simulink model "snb_d"  (R2012b)
settings: Solver=FixedStepDiscrete  SolverMode=SingleTasking  StartTime=0.0  StopTime=10000  RelTol=1e-3
undefined symbols (not defined in the file): Down, pfb_coeff_gen_calc, Up, xlipgetpartsetting
libraries: xbsIndex_r4 x12106, casper_library_misc x14, casper_library_communications x8, casper_library_delays x1, xps_library x1
(part 20 of 79)

== system snb_d/ct/parity_check0 ==
  sync_in : Inport
  din : Inport  Port=2
  en : Inport  Port=3
  Delay : xbsIndex_r4/Delay  rst=off  infoeditControl=Selection of Reset will increase slice count due to use of real FFs and instead of SRLs  en=off  latency=1  dbl_ovrd=off  reg_retiming=on  block_type=delay
  Delay1 : xbsIndex_r4/Delay  rst=off  infoeditControl=Selection of Reset will increase slice count due to use of real FFs and instead of SRLs  en=off  latency=1  dbl_ovrd=off  reg_retiming=on  block_type=delay
  Delay2 : xbsIndex_r4/Delay  rst=off  infoeditControl=Selection of Reset will increase slice count due to use of real FFs and instead of SRLs  en=off  latency=1  dbl_ovrd=off  reg_retiming=on  block_type=delay
  Slice : xbsIndex_r4/Slice  nbits=64  boolean_output=off  mode=Lower Bit Location + Width  bit1=0  base1=MSB of Input  bit0=0  base0=LSB of Input  dbl_ovrd=off  block_type=slice
  Slice1 : xbsIndex_r4/Slice  nbits=1  boolean_output=off  mode=Upper Bit Location + Width  bit1=0  base1=MSB of Input  bit0=0  base0=LSB of Input  dbl_ovrd=off  block_type=slice
  bus_expand : Subsystem  AncestorBlock=casper_library_flow_control/bus_expand  mask(bus_expand){mode=divisions of equal size, outputNum=72, outputWidth=1, outputBinaryPt=0, outputArithmeticType=0, show_format=off, outputToWorkspace=off, variablePrefix=out, outputToModelAsWell=on}
      mask prompts: outputNum "Number of outputs:"; outputWidth "Output width:"; outputBinaryPt "Output binary point position:"; outputArithmeticType "Output arithmetic type (ufix=0, fix=1, bool=2):"; show_format "Print format string?"; outputToWorkspace "Output to workspace?"; variablePrefix "Variable name prefix:"; outputToModelAsWell "Output to model as well?"
      mask help:
      | Expands a 'bus' made using a bus_create or Xilinx
      | concat block.
      | The input will be divided into the specified number
      | of outputs with the specified arithmetic types.
      | Divisions are made from most significant bit.
      mask init: same as snb_d/bus_expand10
      settings: AttributesFormatString=72 outputs
      mask TypeOptions mode: divisions of equal size | divisions of arbitrary size
      mask Callback mode: bus_expand_callback();
      mask Callback outputWidth: bus_expand_callback();
      mask Callback outputToWorkspace: bus_expand_callback();
  parity : xbsIndex_r4/Logical  logical_function=XOR  inputs=72  en=off  latency=1  precision=Full  arith_type=Unsigned  n_bits=16  bin_pt=0  align_bp=on  dbl_ovrd=off  block_type=logical
  parity_error : xbsIndex_r4/Logical  logical_function=AND  inputs=2  en=off  latency=0  precision=Full  arith_type=Unsigned  n_bits=16  bin_pt=0  align_bp=on  dbl_ovrd=off  block_type=logical
  sync_out : Outport
  dout : Outport  Port=2
  dvalid : Outport  Port=3
  error : Outport  Port=4
  wires:
  Slice/1 -> dout/1
  parity_error/1 -> error/1
  parity/1 -> parity_error/1
  sync_in/1 -> Delay/1
  bus_expand/17(out56) -> parity/17
  bus_expand/9(out64) -> parity/9
  bus_expand/64(out9) -> parity/64
  bus_expand/25(out48) -> parity/25
  bus_expand/30(out43) -> parity/30
  bus_expand/39(out34) -> parity/39
  bus_expand/15(out58) -> parity/15
  bus_expand/23(out50) -> parity/23
  bus_expand/16(out57) -> parity/16
  bus_expand/56(out17) -> parity/56
  bus_expand/43(out30) -> parity/43
  bus_expand/34(out39) -> parity/34
  bus_expand/33(out40) -> parity/33
  bus_expand/55(out18) -> parity/55
  bus_expand/29(out44) -> parity/29
  bus_expand/42(out31) -> parity/42
  bus_expand/65(out8) -> parity/65
  bus_expand/10(out63) -> parity/10
  bus_expand/31(out42) -> parity/31
  bus_expand/6(out67) -> parity/6
  bus_expand/1(msb_out72) -> parity/1
  bus_expand/24(out49) -> parity/24
  bus_expand/28(out45) -> parity/28
  bus_expand/47(out26) -> parity/47
  bus_expand/63(out10) -> parity/63
  bus_expand/40(out33) -> parity/40
  bus_expand/20(out53) -> parity/20
  bus_expand/67(out6) -> parity/67
  bus_expand/72(lsb_out1) -> parity/72
  bus_expand/35(out38) -> parity/35
  bus_expand/45(out28) -> parity/45
  bus_expand/32(out41) -> parity/32
  bus_expand/57(out16) -> parity/57
  bus_expand/46(out27) -> parity/46
  bus_expand/38(out35) -> parity/38
  bus_expand/48(out25) -> parity/48
  bus_expand/68(out5) -> parity/68
  bus_expand/7(out66) -> parity/7
  bus_expand/27(out46) -> parity/27
  bus_expand/41(out32) -> parity/41
  bus_expand/62(out11) -> parity/62
  bus_expand/3(out70) -> parity/3
  bus_expand/70(out3) -> parity/70
  bus_expand/4(out69) -> parity/4
  bus_expand/37(out36) -> parity/37
  bus_expand/71(out2) -> parity/71
  bus_expand/19(out54) -> parity/19
  bus_expand/66(out7) -> parity/66
  bus_expand/8(out65) -> parity/8
  bus_expand/49(out24) -> parity/49
  bus_expand/50(out23) -> parity/50
  bus_expand/21(out52) -> parity/21
  bus_expand/60(out13) -> parity/60
  bus_expand/59(out14) -> parity/59
  bus_expand/12(out61) -> parity/12
  bus_expand/53(out20) -> parity/53
  bus_expand/69(out4) -> parity/69
  bus_expand/36(out37) -> parity/36
  bus_expand/13(out60) -> parity/13
  bus_expand/26(out47) -> parity/26
  bus_expand/51(out22) -> parity/51
  bus_expand/58(out15) -> parity/58
  bus_expand/61(out12) -> parity/61
  bus_expand/5(out68) -> parity/5
  bus_expand/44(out29) -> parity/44
  bus_expand/54(out19) -> parity/54
  bus_expand/18(out55) -> parity/18
  bus_expand/2(out71) -> parity/2
  bus_expand/22(out51) -> parity/22
  bus_expand/52(out21) -> parity/52
  bus_expand/14(out59) -> parity/14
  bus_expand/11(out62) -> parity/11
  Delay1/1 -> Slice/1
  en/1 -> Delay2/1
  Delay/1 -> sync_out/1
  din/1 -> bus_expand/1(bus_in), Delay1/1
  Delay2/1 -> dvalid/1, Slice1/1
  Slice1/1 -> parity_error/2

== system snb_d/ct/parity_check1 ==
  sync_in : Inport
  din : Inport  Port=2
  en : Inport  Port=3
  Delay : xbsIndex_r4/Delay  rst=off  infoeditControl=Selection of Reset will increase slice count due to use of real FFs and instead of SRLs  en=off  latency=1  dbl_ovrd=off  reg_retiming=on  block_type=delay
  Delay1 : xbsIndex_r4/Delay  rst=off  infoeditControl=Selection of Reset will increase slice count due to use of real FFs and instead of SRLs  en=off  latency=1  dbl_ovrd=off  reg_retiming=on  block_type=delay
  Delay2 : xbsIndex_r4/Delay  rst=off  infoeditControl=Selection of Reset will increase slice count due to use of real FFs and instead of SRLs  en=off  latency=1  dbl_ovrd=off  reg_retiming=on  block_type=delay
  Slice : xbsIndex_r4/Slice  nbits=64  boolean_output=off  mode=Lower Bit Location + Width  bit1=0  base1=MSB of Input  bit0=0  base0=LSB of Input  dbl_ovrd=off  block_type=slice
  Slice1 : xbsIndex_r4/Slice  nbits=1  boolean_output=off  mode=Upper Bit Location + Width  bit1=0  base1=MSB of Input  bit0=0  base0=LSB of Input  dbl_ovrd=off  block_type=slice
  bus_expand : Subsystem  AncestorBlock=casper_library_flow_control/bus_expand  mask(bus_expand){mode=divisions of equal size, outputNum=72, outputWidth=1, outputBinaryPt=0, outputArithmeticType=0, show_format=off, outputToWorkspace=off, variablePrefix=out, outputToModelAsWell=on}
      mask prompts: outputNum "Number of outputs:"; outputWidth "Output width:"; outputBinaryPt "Output binary point position:"; outputArithmeticType "Output arithmetic type (ufix=0, fix=1, bool=2):"; show_format "Print format string?"; outputToWorkspace "Output to workspace?"; variablePrefix "Variable name prefix:"; outputToModelAsWell "Output to model as well?"
      mask help:
      | Expands a 'bus' made using a bus_create or Xilinx
      | concat block.
      | The input will be divided into the specified number
      | of outputs with the specified arithmetic types.
      | Divisions are made from most significant bit.
      mask init: same as snb_d/bus_expand10
      settings: AttributesFormatString=72 outputs
      mask TypeOptions mode: divisions of equal size | divisions of arbitrary size
      mask Callback mode: bus_expand_callback();
      mask Callback outputWidth: bus_expand_callback();
      mask Callback outputToWorkspace: bus_expand_callback();
  parity : xbsIndex_r4/Logical  logical_function=XOR  inputs=72  en=off  latency=1  precision=Full  arith_type=Unsigned  n_bits=16  bin_pt=0  align_bp=on  dbl_ovrd=off  block_type=logical
  parity_error : xbsIndex_r4/Logical  logical_function=AND  inputs=2  en=off  latency=0  precision=Full  arith_type=Unsigned  n_bits=16  bin_pt=0  align_bp=on  dbl_ovrd=off  block_type=logical
  sync_out : Outport
  dout : Outport  Port=2
  dvalid : Outport  Port=3
  error : Outport  Port=4
  wires:
  Slice1/1 -> parity_error/2
  Delay2/1 -> Slice1/1, dvalid/1
  din/1 -> Delay1/1, bus_expand/1(bus_in)
  Delay/1 -> sync_out/1
  en/1 -> Delay2/1
  Delay1/1 -> Slice/1
  bus_expand/11(out62) -> parity/11
  bus_expand/14(out59) -> parity/14
  bus_expand/52(out21) -> parity/52
  bus_expand/22(out51) -> parity/22
  bus_expand/2(out71) -> parity/2
  bus_expand/18(out55) -> parity/18
  bus_expand/54(out19) -> parity/54
  bus_expand/44(out29) -> parity/44
  bus_expand/5(out68) -> parity/5
  bus_expand/61(out12) -> parity/61
  bus_expand/58(out15) -> parity/58
  bus_expand/51(out22) -> parity/51
  bus_expand/26(out47) -> parity/26
  bus_expand/13(out60) -> parity/13
  bus_expand/36(out37) -> parity/36
  bus_expand/69(out4) -> parity/69
  bus_expand/53(out20) -> parity/53
  bus_expand/12(out61) -> parity/12
  bus_expand/59(out14) -> parity/59
  bus_expand/60(out13) -> parity/60
  bus_expand/21(out52) -> parity/21
  bus_expand/50(out23) -> parity/50
  bus_expand/49(out24) -> parity/49
  bus_expand/8(out65) -> parity/8
  bus_expand/66(out7) -> parity/66
  bus_expand/19(out54) -> parity/19
  bus_expand/71(out2) -> parity/71
  bus_expand/37(out36) -> parity/37
  bus_expand/4(out69) -> parity/4
  bus_expand/70(out3) -> parity/70
  bus_expand/3(out70) -> parity/3
  bus_expand/62(out11) -> parity/62
  bus_expand/41(out32) -> parity/41
  bus_expand/27(out46) -> parity/27
  bus_expand/7(out66) -> parity/7
  bus_expand/68(out5) -> parity/68
  bus_expand/48(out25) -> parity/48
  bus_expand/38(out35) -> parity/38
  bus_expand/46(out27) -> parity/46
  bus_expand/57(out16) -> parity/57
  bus_expand/32(out41) -> parity/32
  bus_expand/45(out28) -> parity/45
  bus_expand/35(out38) -> parity/35
  bus_expand/72(lsb_out1) -> parity/72
  bus_expand/67(out6) -> parity/67
  bus_expand/20(out53) -> parity/20
  bus_expand/40(out33) -> parity/40
  bus_expand/63(out10) -> parity/63
  bus_expand/47(out26) -> parity/47
  bus_expand/28(out45) -> parity/28
  bus_expand/24(out49) -> parity/24
  bus_expand/1(msb_out72) -> parity/1
  bus_expand/6(out67) -> parity/6
  bus_expand/31(out42) -> parity/31
  bus_expand/10(out63) -> parity/10
  bus_expand/65(out8) -> parity/65
  bus_expand/42(out31) -> parity/42
  bus_expand/29(out44) -> parity/29
  bus_expand/55(out18) -> parity/55
  bus_expand/33(out40) -> parity/33
  bus_expand/34(out39) -> parity/34
  bus_expand/43(out30) -> parity/43
  bus_expand/56(out17) -> parity/56
  bus_expand/16(out57) -> parity/16
  bus_expand/23(out50) -> parity/23
  bus_expand/15(out58) -> parity/15
  bus_expand/39(out34) -> parity/39
  bus_expand/30(out43) -> parity/30
  bus_expand/25(out48) -> parity/25
  bus_expand/64(out9) -> parity/64
  bus_expand/9(out64) -> parity/9
  bus_expand/17(out56) -> parity/17
  sync_in/1 -> Delay/1
  parity/1 -> parity_error/1
  parity_error/1 -> error/1
  Slice/1 -> dout/1

== system snb_d/ct/parity_generation0 ==
  sync_in : Inport
  din : Inport  Port=2
  en : Inport  Port=3
  Concat : xbsIndex_r4/Concat  num_inputs=3  dbl_ovrd=off  block_type=concat
  Delay : xbsIndex_r4/Delay  rst=off  infoeditControl=Selection of Reset will increase slice count due to use of real FFs and instead of SRLs  en=off  latency=1  dbl_ovrd=off  reg_retiming=on  block_type=delay
  Delay1 : xbsIndex_r4/Delay  rst=off  infoeditControl=Selection of Reset will increase slice count due to use of real FFs and instead of SRLs  en=off  latency=1  dbl_ovrd=off  reg_retiming=on  block_type=delay
  Delay2 : xbsIndex_r4/Delay  rst=off  infoeditControl=Selection of Reset will increase slice count due to use of real FFs and instead of SRLs  en=off  latency=1  dbl_ovrd=off  reg_retiming=on  block_type=delay
  bus_expand : Subsystem  AncestorBlock=casper_library_flow_control/bus_expand  mask(bus_expand){mode=divisions of equal size, outputNum=64, outputWidth=1, outputBinaryPt=0, outputArithmeticType=0, show_format=off, outputToWorkspace=off, variablePrefix=out, outputToModelAsWell=on}
      mask prompts: outputNum "Number of outputs:"; outputWidth "Output width:"; outputBinaryPt "Output binary point position:"; outputArithmeticType "Output arithmetic type (ufix=0, fix=1, bool=2):"; show_format "Print format string?"; outputToWorkspace "Output to workspace?"; variablePrefix "Variable name prefix:"; outputToModelAsWell "Output to model as well?"
      mask help:
      | Expands a 'bus' made using a bus_create or Xilinx
      | concat block.
      | The input will be divided into the specified number
      | of outputs with the specified arithmetic types.
      | Divisions are made from most significant bit.
      mask init: same as snb_d/bus_expand10
      settings: AttributesFormatString=64 outputs
      mask TypeOptions mode: divisions of equal size | divisions of arbitrary size
      mask Callback mode: bus_expand_callback();
      mask Callback outputWidth: bus_expand_callback();
      mask Callback outputToWorkspace: bus_expand_callback();
  padding : xbsIndex_r4/Constant  const=0  gui_display_data_type=Fixed-point  arith_type=Unsigned  n_bits=72-64-1  bin_pt=0  preci_type=Single  exp_width=8  frac_width=24  explicit_period=on  period=1  equ=P=C  opselect=C  inp2=PCIN>>17  opr=+  inp1=P  carry=CIN  dbl_ovrd=off  block_type=constant
  parity : xbsIndex_r4/Logical  logical_function=XOR  inputs=64  en=off  latency=1  precision=Full  arith_type=Unsigned  n_bits=16  bin_pt=0  align_bp=on  dbl_ovrd=off  block_type=logical
  sync_out : Outport
  dout : Outport  Port=2
  dvalid : Outport  Port=3
  wires:
  padding/1 -> Concat/2
  Delay2/1 -> dvalid/1
  Concat/1 -> dout/1
  parity/1 -> Concat/1
  Delay1/1 -> Concat/3
  en/1 -> Delay2/1
  din/1 -> Delay1/1, bus_expand/1(bus_in)
  Delay/1 -> sync_out/1
  sync_in/1 -> Delay/1
  bus_expand/33(out32) -> parity/33
  bus_expand/14(out51) -> parity/14
  bus_expand/9(out56) -> parity/9
  bus_expand/47(out18) -> parity/47
  bus_expand/59(out6) -> parity/59
  bus_expand/43(out22) -> parity/43
  bus_expand/40(out25) -> parity/40
  bus_expand/38(out27) -> parity/38
  bus_expand/18(out47) -> parity/18
  bus_expand/21(out44) -> parity/21
  bus_expand/1(msb_out64) -> parity/1
  bus_expand/3(out62) -> parity/3
  bus_expand/16(out49) -> parity/16
  bus_expand/64(lsb_out1) -> parity/64
  bus_expand/60(out5) -> parity/60
  bus_expand/39(out26) -> parity/39
  bus_expand/30(out35) -> parity/30
  bus_expand/44(out21) -> parity/44
  bus_expand/56(out9) -> parity/56
  bus_expand/28(out37) -> parity/28
  bus_expand/53(out12) -> parity/53
  bus_expand/4(out61) -> parity/4
  bus_expand/62(out3) -> parity/62
  bus_expand/10(out55) -> parity/10
  bus_expand/48(out17) -> parity/48
  bus_expand/31(out34) -> parity/31
  bus_expand/17(out48) -> parity/17
  bus_expand/54(out11) -> parity/54
  bus_expand/51(out14) -> parity/51
  bus_expand/57(out8) -> parity/57
  bus_expand/22(out43) -> parity/22
  bus_expand/35(out30) -> parity/35
  bus_expand/50(out15) -> parity/50
  bus_expand/55(out10) -> parity/55
  bus_expand/32(out33) -> parity/32
  bus_expand/36(out29) -> parity/36
  bus_expand/20(out45) -> parity/20
  bus_expand/26(out39) -> parity/26
  bus_expand/7(out58) -> parity/7
  bus_expand/12(out53) -> parity/12
  bus_expand/23(out42) -> parity/23
  bus_expand/2(out63) -> parity/2
  bus_expand/19(out46) -> parity/19
  bus_expand/61(out4) -> parity/61
  bus_expand/29(out36) -> parity/29
  bus_expand/25(out40) -> parity/25
  bus_expand/15(out50) -> parity/15
  bus_expand/46(out19) -> parity/46
  bus_expand/52(out13) -> parity/52
  bus_expand/34(out31) -> parity/34
  bus_expand/63(out2) -> parity/63
  bus_expand/58(out7) -> parity/58
  bus_expand/24(out41) -> parity/24
  bus_expand/6(out59) -> parity/6
  bus_expand/13(out52) -> parity/13
  bus_expand/27(out38) -> parity/27
  bus_expand/45(out20) -> parity/45
  bus_expand/37(out28) -> parity/37
  bus_expand/5(out60) -> parity/5
  bus_expand/11(out54) -> parity/11
  bus_expand/49(out16) -> parity/49
  bus_expand/42(out23) -> parity/42
  bus_expand/41(out24) -> parity/41
  bus_expand/8(out57) -> parity/8

== system snb_d/ct/parity_generation1 ==
  sync_in : Inport
  din : Inport  Port=2
  en : Inport  Port=3
  Concat : xbsIndex_r4/Concat  num_inputs=3  dbl_ovrd=off  block_type=concat
  Delay : xbsIndex_r4/Delay  rst=off  infoeditControl=Selection of Reset will increase slice count due to use of real FFs and instead of SRLs  en=off  latency=1  dbl_ovrd=off  reg_retiming=on  block_type=delay
  Delay1 : xbsIndex_r4/Delay  rst=off  infoeditControl=Selection of Reset will increase slice count due to use of real FFs and instead of SRLs  en=off  latency=1  dbl_ovrd=off  reg_retiming=on  block_type=delay
  Delay2 : xbsIndex_r4/Delay  rst=off  infoeditControl=Selection of Reset will increase slice count due to use of real FFs and instead of SRLs  en=off  latency=1  dbl_ovrd=off  reg_retiming=on  block_type=delay
  bus_expand : Subsystem  AncestorBlock=casper_library_flow_control/bus_expand  mask(bus_expand){mode=divisions of equal size, outputNum=64, outputWidth=1, outputBinaryPt=0, outputArithmeticType=0, show_format=off, outputToWorkspace=off, variablePrefix=out, outputToModelAsWell=on}
      mask prompts: outputNum "Number of outputs:"; outputWidth "Output width:"; outputBinaryPt "Output binary point position:"; outputArithmeticType "Output arithmetic type (ufix=0, fix=1, bool=2):"; show_format "Print format string?"; outputToWorkspace "Output to workspace?"; variablePrefix "Variable name prefix:"; outputToModelAsWell "Output to model as well?"
      mask help:
      | Expands a 'bus' made using a bus_create or Xilinx
      | concat block.
      | The input will be divided into the specified number
      | of outputs with the specified arithmetic types.
      | Divisions are made from most significant bit.
      mask init: same as snb_d/bus_expand10
      settings: AttributesFormatString=64 outputs
      mask TypeOptions mode: divisions of equal size | divisions of arbitrary size
      mask Callback mode: bus_expand_callback();
      mask Callback outputWidth: bus_expand_callback();
      mask Callback outputToWorkspace: bus_expand_callback();
  padding : xbsIndex_r4/Constant  const=0  gui_display_data_type=Fixed-point  arith_type=Unsigned  n_bits=72-64-1  bin_pt=0  preci_type=Single  exp_width=8  frac_width=24  explicit_period=on  period=1  equ=P=C  opselect=C  inp2=PCIN>>17  opr=+  inp1=P  carry=CIN  dbl_ovrd=off  block_type=constant
  parity : xbsIndex_r4/Logical  logical_function=XOR  inputs=64  en=off  latency=1  precision=Full  arith_type=Unsigned  n_bits=16  bin_pt=0  align_bp=on  dbl_ovrd=off  block_type=logical
  sync_out : Outport
  dout : Outport  Port=2
  dvalid : Outport  Port=3
  wires:
  bus_expand/8(out57) -> parity/8
  bus_expand/41(out24) -> parity/41
  bus_expand/42(out23) -> parity/42
  bus_expand/49(out16) -> parity/49
  bus_expand/11(out54) -> parity/11
  bus_expand/5(out60) -> parity/5
  bus_expand/37(out28) -> parity/37
  bus_expand/45(out20) -> parity/45
  bus_expand/27(out38) -> parity/27
  bus_expand/13(out52) -> parity/13
  bus_expand/6(out59) -> parity/6
  bus_expand/24(out41) -> parity/24
  bus_expand/58(out7) -> parity/58
  bus_expand/63(out2) -> parity/63
  bus_expand/34(out31) -> parity/34
  bus_expand/52(out13) -> parity/52
  bus_expand/46(out19) -> parity/46
  bus_expand/15(out50) -> parity/15
  bus_expand/25(out40) -> parity/25
  bus_expand/29(out36) -> parity/29
  bus_expand/61(out4) -> parity/61
  bus_expand/19(out46) -> parity/19
  bus_expand/2(out63) -> parity/2
  bus_expand/23(out42) -> parity/23
  bus_expand/12(out53) -> parity/12
  bus_expand/7(out58) -> parity/7
  bus_expand/26(out39) -> parity/26
  bus_expand/20(out45) -> parity/20
  bus_expand/36(out29) -> parity/36
  bus_expand/32(out33) -> parity/32
  bus_expand/55(out10) -> parity/55
  bus_expand/50(out15) -> parity/50
  bus_expand/35(out30) -> parity/35
  bus_expand/22(out43) -> parity/22
  bus_expand/57(out8) -> parity/57
  bus_expand/51(out14) -> parity/51
  bus_expand/54(out11) -> parity/54
  bus_expand/17(out48) -> parity/17
  bus_expand/31(out34) -> parity/31
  bus_expand/48(out17) -> parity/48
  bus_expand/10(out55) -> parity/10
  bus_expand/62(out3) -> parity/62
  bus_expand/4(out61) -> parity/4
  bus_expand/53(out12) -> parity/53
  bus_expand/28(out37) -> parity/28
  bus_expand/56(out9) -> parity/56
  bus_expand/44(out21) -> parity/44
  bus_expand/30(out35) -> parity/30
  bus_expand/39(out26) -> parity/39
  bus_expand/60(out5) -> parity/60
  bus_expand/64(lsb_out1) -> parity/64
  bus_expand/16(out49) -> parity/16
  bus_expand/3(out62) -> parity/3
  bus_expand/1(msb_out64) -> parity/1
  bus_expand/21(out44) -> parity/21
  bus_expand/18(out47) -> parity/18
  bus_expand/38(out27) -> parity/38
  bus_expand/40(out25) -> parity/40
  bus_expand/43(out22) -> parity/43
  bus_expand/59(out6) -> parity/59
  bus_expand/47(out18) -> parity/47
  bus_expand/9(out56) -> parity/9
  bus_expand/14(out51) -> parity/14
  bus_expand/33(out32) -> parity/33
  sync_in/1 -> Delay/1
  Delay/1 -> sync_out/1
  din/1 -> bus_expand/1(bus_in), Delay1/1
  en/1 -> Delay2/1
  Delay1/1 -> Concat/3
  parity/1 -> Concat/1
  Concat/1 -> dout/1
  Delay2/1 -> dvalid/1
  padding/1 -> Concat/2

== system snb_d/ct/pipeline ==
  d : Inport
  Register0 : xbsIndex_r4/Register  init=0  rst=off  en=off  dbl_ovrd=off  block_type=register
      settings: block_version=11.4
  Register1 : xbsIndex_r4/Register  init=0  rst=off  en=off  dbl_ovrd=off  block_type=register
      settings: block_version=11.4
  Register2 : xbsIndex_r4/Register  init=0  rst=off  en=off  dbl_ovrd=off  block_type=register
  q : Outport
  wires:
  Register0/1 -> Register1/1
  Register1/1 -> Register2/1
  d/1 -> Register0/1
  Register2/1 -> q/1

== system snb_d/ct/pipeline1 ==
  d : Inport
  Register0 : xbsIndex_r4/Register  init=0  rst=off  en=off  dbl_ovrd=off  block_type=register
      settings: block_version=11.4
  Register1 : xbsIndex_r4/Register  init=0  rst=off  en=off  dbl_ovrd=off  block_type=register
      settings: block_version=11.4
  Register2 : xbsIndex_r4/Register  init=0  rst=off  en=off  dbl_ovrd=off  block_type=register
  q : Outport
  wires:
  Register2/1 -> q/1
  d/1 -> Register0/1
  Register1/1 -> Register2/1
  Register0/1 -> Register1/1

== system snb_d/ct/pipeline10 ==
  d : Inport
  Register0 : xbsIndex_r4/Register  init=0  rst=off  en=off  dbl_ovrd=off  block_type=register
      settings: block_version=11.4
  Register1 : xbsIndex_r4/Register  init=0  rst=off  en=off  dbl_ovrd=off  block_type=register
      settings: block_version=11.4
  Register2 : xbsIndex_r4/Register  init=0  rst=off  en=off  dbl_ovrd=off  block_type=register
  q : Outport
  wires:
  Register0/1 -> Register1/1
  Register1/1 -> Register2/1
  d/1 -> Register0/1
  Register2/1 -> q/1

== system snb_d/ct/pipeline11 ==
  d : Inport
  Register0 : xbsIndex_r4/Register  init=0  rst=off  en=off  dbl_ovrd=off  block_type=register
      settings: block_version=11.4
  Register1 : xbsIndex_r4/Register  init=0  rst=off  en=off  dbl_ovrd=off  block_type=register
      settings: block_version=11.4
  Register2 : xbsIndex_r4/Register  init=0  rst=off  en=off  dbl_ovrd=off  block_type=register
  q : Outport
  wires:
  Register2/1 -> q/1
  d/1 -> Register0/1
  Register1/1 -> Register2/1
  Register0/1 -> Register1/1

== system snb_d/ct/pipeline12 ==
  d : Inport
  Register0 : xbsIndex_r4/Register  init=0  rst=off  en=off  dbl_ovrd=off  block_type=register
      settings: block_version=11.4
  Register1 : xbsIndex_r4/Register  init=0  rst=off  en=off  dbl_ovrd=off  block_type=register
      settings: block_version=11.4
  Register2 : xbsIndex_r4/Register  init=0  rst=off  en=off  dbl_ovrd=off  block_type=register
  q : Outport
  wires:
  Register0/1 -> Register1/1
  Register1/1 -> Register2/1
  d/1 -> Register0/1
  Register2/1 -> q/1

== system snb_d/ct/pipeline13 ==
  d : Inport
  Register0 : xbsIndex_r4/Register  init=0  rst=off  en=off  dbl_ovrd=off  block_type=register
      settings: block_version=11.4
  Register1 : xbsIndex_r4/Register  init=0  rst=off  en=off  dbl_ovrd=off  block_type=register
      settings: block_version=11.4
  Register2 : xbsIndex_r4/Register  init=0  rst=off  en=off  dbl_ovrd=off  block_type=register
  q : Outport
  wires:
  Register2/1 -> q/1
  d/1 -> Register0/1
  Register1/1 -> Register2/1
  Register0/1 -> Register1/1

== system snb_d/ct/pipeline2 ==
  d : Inport
  Register0 : xbsIndex_r4/Register  init=0  rst=off  en=off  dbl_ovrd=off  block_type=register
      settings: block_version=11.4
  Register1 : xbsIndex_r4/Register  init=0  rst=off  en=off  dbl_ovrd=off  block_type=register
      settings: block_version=11.4
  Register2 : xbsIndex_r4/Register  init=0  rst=off  en=off  dbl_ovrd=off  block_type=register
  q : Outport
  wires:
  Register0/1 -> Register1/1
  Register1/1 -> Register2/1
  d/1 -> Register0/1
  Register2/1 -> q/1

== system snb_d/ct/pipeline3 ==
  d : Inport
  Register0 : xbsIndex_r4/Register  init=0  rst=off  en=off  dbl_ovrd=off  block_type=register
      settings: block_version=11.4
  Register1 : xbsIndex_r4/Register  init=0  rst=off  en=off  dbl_ovrd=off  block_type=register
      settings: block_version=11.4
  Register2 : xbsIndex_r4/Register  init=0  rst=off  en=off  dbl_ovrd=off  block_type=register
  q : Outport
  wires:
  Register2/1 -> q/1
  d/1 -> Register0/1
  Register1/1 -> Register2/1
  Register0/1 -> Register1/1

== system snb_d/ct/pipeline4 ==
  d : Inport
  Register0 : xbsIndex_r4/Register  init=0  rst=off  en=off  dbl_ovrd=off  block_type=register
      settings: block_version=11.4
  Register1 : xbsIndex_r4/Register  init=0  rst=off  en=off  dbl_ovrd=off  block_type=register
      settings: block_version=11.4
  Register2 : xbsIndex_r4/Register  init=0  rst=off  en=off  dbl_ovrd=off  block_type=register
  q : Outport
  wires:
  Register0/1 -> Register1/1
  Register1/1 -> Register2/1
  d/1 -> Register0/1
  Register2/1 -> q/1

== system snb_d/ct/pipeline5 ==
  d : Inport
  Register0 : xbsIndex_r4/Register  init=0  rst=off  en=off  dbl_ovrd=off  block_type=register
      settings: block_version=11.4
  Register1 : xbsIndex_r4/Register  init=0  rst=off  en=off  dbl_ovrd=off  block_type=register
      settings: block_version=11.4
  Register2 : xbsIndex_r4/Register  init=0  rst=off  en=off  dbl_ovrd=off  block_type=register
  q : Outport
  wires:
  Register2/1 -> q/1
  d/1 -> Register0/1
  Register1/1 -> Register2/1
  Register0/1 -> Register1/1

== system snb_d/ct/pipeline6 ==
  d : Inport
  Register0 : xbsIndex_r4/Register  init=0  rst=off  en=off  dbl_ovrd=off  block_type=register
      settings: block_version=11.4
  Register1 : xbsIndex_r4/Register  init=0  rst=off  en=off  dbl_ovrd=off  block_type=register
      settings: block_version=11.4
  Register2 : xbsIndex_r4/Register  init=0  rst=off  en=off  dbl_ovrd=off  block_type=register
  q : Outport
  wires:
  Register0/1 -> Register1/1
  Register1/1 -> Register2/1
  d/1 -> Register0/1
  Register2/1 -> q/1

== system snb_d/ct/pipeline7 ==
  d : Inport
  Register0 : xbsIndex_r4/Register  init=0  rst=off  en=off  dbl_ovrd=off  block_type=register
      settings: block_version=11.4
  Register1 : xbsIndex_r4/Register  init=0  rst=off  en=off  dbl_ovrd=off  block_type=register
      settings: block_version=11.4
  Register2 : xbsIndex_r4/Register  init=0  rst=off  en=off  dbl_ovrd=off  block_type=register
  q : Outport
  wires:
  Register2/1 -> q/1
  d/1 -> Register0/1
  Register1/1 -> Register2/1
  Register0/1 -> Register1/1

== system snb_d/ct/pipeline8 ==
  d : Inport
  Register0 : xbsIndex_r4/Register  init=0  rst=off  en=off  dbl_ovrd=off  block_type=register
      settings: block_version=11.4
  Register1 : xbsIndex_r4/Register  init=0  rst=off  en=off  dbl_ovrd=off  block_type=register
      settings: block_version=11.4
  Register2 : xbsIndex_r4/Register  init=0  rst=off  en=off  dbl_ovrd=off  block_type=register
  q : Outport
  wires:
  Register0/1 -> Register1/1
  Register1/1 -> Register2/1
  d/1 -> Register0/1
  Register2/1 -> q/1

== system snb_d/ct/pipeline9 ==
  d : Inport
  Register0 : xbsIndex_r4/Register  init=0  rst=off  en=off  dbl_ovrd=off  block_type=register
      settings: block_version=11.4
  Register1 : xbsIndex_r4/Register  init=0  rst=off  en=off  dbl_ovrd=off  block_type=register
      settings: block_version=11.4
  Register2 : xbsIndex_r4/Register  init=0  rst=off  en=off  dbl_ovrd=off  block_type=register
  q : Outport
  wires:
  Register2/1 -> q/1
  d/1 -> Register0/1
  Register1/1 -> Register2/1
  Register0/1 -> Register1/1

== system snb_d/ct/qdr_ct_nobram0 ==
  note: Write control
  note: The eight cycles after a write are valid read cycles.
      | That's four QDR reads.
  note: Reads are only armed after a sync and after the first write.
  note: A read cycle begins after writing past the halfway mark of
      | the address range.
  note: Read enable signal is a combination of enables and arms.
  note: Counter to track where in the read process we are.
  note: After reading one packet-worth of data, we pause for a period.
  note: Change the read address
      | on alternate read cycles
      | (double buffered).
  note: Only need input_bits + ct_bits as two words are
      | written per address in QDR. So double-buffering
      | is done.
  note: Doing it manually to save BRAM.
  in_sync : Inport
  in_dv : Inport  Port=2
  in_data64 : Inport  Port=3
  ct_reset : Inport  Port=4
  AddSub : xbsIndex_r4/AddSub  mode=Addition  use_carryin=off  use_carryout=off  en=off  latency=0  precision=User Defined  arith_type=Unsigned  n_bits=input_bits + ct_bits - 1  bin_pt=0  quantization=Truncate  overflow=Wrap  dbl_ovrd=off  use_behavioral_HDL=on  hw_selection=Fabric  pipelined=off  block_type=addsub
  AddSub1 : xbsIndex_r4/AddSub  mode=Addition  use_carryin=off  use_carryout=off  en=off  latency=0  precision=User Defined  arith_type=Unsigned  n_bits=input_bits + ct_bits - 1  bin_pt=0  quantization=Truncate  overflow=Wrap  dbl_ovrd=off  use_behavioral_HDL=on  hw_selection=Fabric  pipelined=off  block_type=addsub
  Concat2 : xbsIndex_r4/Concat  num_inputs=2  dbl_ovrd=off  block_type=concat
  Concat3 : xbsIndex_r4/Concat  num_inputs=2  dbl_ovrd=off  block_type=concat
  Concat4 : xbsIndex_r4/Concat  num_inputs=2  dbl_ovrd=off  block_type=concat
  Constant : xbsIndex_r4/Constant  const=0  gui_display_data_type=Fixed-point  arith_type=Unsigned  n_bits=input_bits - x_bits - 1  bin_pt=0  preci_type=Single  exp_width=8  frac_width=24  explicit_period=on  period=1  equ=P=C  opselect=C  inp2=PCIN>>17  opr=+  inp1=P  carry=CIN  dbl_ovrd=off  block_type=constant
  Constant2 : xbsIndex_r4/Constant  const=1  gui_display_data_type=Boolean  arith_type=Boolean  n_bits=4  bin_pt=0  preci_type=Single  exp_width=8  frac_width=24  explicit_period=on  period=1  equ=P=C  opselect=C  inp2=PCIN>>17  opr=+  inp1=P  carry=CIN  dbl_ovrd=off  block_type=constant
  Constant5 : xbsIndex_r4/Constant  const=15  gui_display_data_type=Fixed-point  arith_type=Unsigned  n_bits=4  bin_pt=0  preci_type=Single  exp_width=8  frac_width=24  explicit_period=on  period=1  equ=P=C  opselect=C  inp2=PCIN>>17  opr=+  inp1=P  carry=CIN  dbl_ovrd=off  block_type=constant
  Delay{,6..9,14..18} (10 alike) : xbsIndex_r4/Delay  rst=off  infoeditControl=Selection of Reset will increase slice count due to use of real FFs and instead of SRLs  en=off  latency=1  dbl_ovrd=off  reg_retiming=off  block_type=delay
  Delay1 : xbsIndex_r4/Delay  rst=off  infoeditControl=Selection of Reset will increase slice count due to use of real FFs and instead of SRLs  en=off  latency=3  dbl_ovrd=off  reg_retiming=off  block_type=delay
  Delay10 : xbsIndex_r4/Delay  rst=off  infoeditControl=Selection of Reset will increase slice count due to use of real FFs and instead of SRLs  en=off  latency=10  dbl_ovrd=off  reg_retiming=off  block_type=delay
  Delay19 : xbsIndex_r4/Delay  rst=off  infoeditControl=Selection of Reset will increase slice count due to use of real FFs and instead of SRLs  en=off  latency=10  dbl_ovrd=off  reg_retiming=off  block_type=delay
  Delay2 : xbsIndex_r4/Delay  rst=off  infoeditControl=Selection of Reset will increase slice count due to use of real FFs and instead of SRLs  en=off  latency=5  dbl_ovrd=off  reg_retiming=off  block_type=delay
  Delay3 : xbsIndex_r4/Delay  rst=off  infoeditControl=Selection of Reset will increase slice count due to use of real FFs and instead of SRLs  en=off  latency=7  dbl_ovrd=off  reg_retiming=off  block_type=delay
  Delay5 : xbsIndex_r4/Delay  rst=off  infoeditControl=Selection of Reset will increase slice count due to use of real FFs and instead of SRLs  en=off  latency=2  dbl_ovrd=off  reg_retiming=off  block_type=delay
  Inverter : xbsIndex_r4/Inverter  en=off  latency=0  dbl_ovrd=off  block_type=inv
  Logical{,2,4,10} (4 alike) : xbsIndex_r4/Logical  logical_function=OR  inputs=2  en=off  latency=0  precision=Full  arith_type=Unsigned  n_bits=16  bin_pt=0  align_bp=on  dbl_ovrd=off  block_type=logical
  Logical{1,6..9} (5 alike) : xbsIndex_r4/Logical  logical_function=AND  inputs=2  en=off  latency=0  precision=Full  arith_type=Unsigned  n_bits=16  bin_pt=0  align_bp=on  dbl_ovrd=off  block_type=logical
  Logical3 : xbsIndex_r4/Logical  logical_function=OR  inputs=4  en=off  latency=0  precision=Full  arith_type=Unsigned  n_bits=16  bin_pt=0  align_bp=on  dbl_ovrd=off  block_type=logical
  Logical5 : xbsIndex_r4/Logical  logical_function=AND  inputs=4  en=off  latency=0  precision=Full  arith_type=Unsigned  n_bits=16  bin_pt=0  align_bp=on  dbl_ovrd=off  block_type=logical
  Mux1 : xbsIndex_r4/Mux  inputs=2  en=off  latency=0  precision=Full  arith_type=Unsigned  n_bits=16  bin_pt=14  quantization=Truncate  overflow=Wrap  dbl_ovrd=off  block_type=mux
  Mux2 : xbsIndex_r4/Mux  inputs=2  en=off  latency=0  precision=Full  arith_type=Unsigned  n_bits=16  bin_pt=14  quantization=Truncate  overflow=Wrap  dbl_ovrd=off  block_type=mux
  Slice1 : xbsIndex_r4/Slice  nbits=5-1  boolean_output=on  mode=Lower Bit Location + Width  bit1=0  base1=MSB of Input  bit0=ct_bits - 1  base0=LSB of Input  dbl_ovrd=off  block_type=slice
  Slice10 : xbsIndex_r4/Slice  nbits=5-1  boolean_output=on  mode=Lower Bit Location + Width  bit1=0  base1=MSB of Input  bit0=ct_bits + x_bits  base0=LSB of Input  dbl_ovrd=off  block_type=slice
  Slice11 : xbsIndex_r4/Slice  nbits=ct_bits + x_bits  boolean_output=off  mode=Lower Bit Location + Width  bit1=0  base1=MSB of Input  bit0=0  base0=LSB of Input  dbl_ovrd=off  block_type=slice
  Slice12 : xbsIndex_r4/Slice  nbits=input_bits - x_bits - 1  boolean_output=off  mode=Lower Bit Location + Width  bit1=0  base1=MSB of Input  bit0=ct_bits + x_bits + 1  base0=LSB of Input  dbl_ovrd=off  block_type=slice
  Slice2 : xbsIndex_r4/Slice  nbits=5-1  boolean_output=on  mode=Upper Bit Location + Width  bit1=-1  base1=MSB of Input  bit0=input_bits + ct_bits  base0=LSB of Input  dbl_ovrd=off  block_type=slice
  Slice3 : xbsIndex_r4/Slice  nbits=5-1  boolean_output=on  mode=Upper Bit Location + Width  bit1=0  base1=MSB of Input  bit0=2-1  base0=LSB of Input  dbl_ovrd=off  block_type=slice
  Slice4 : xbsIndex_r4/Slice  nbits=x_bits  boolean_output=off  mode=Lower Bit Location + Width  bit1=0  base1=MSB of Input  bit0=ct_bits  base0=LSB of Input  dbl_ovrd=off  block_type=slice
  Slice5 : xbsIndex_r4/Slice  nbits=5-1  boolean_output=on  mode=Upper Bit Location + Width  bit1=0  base1=MSB of Input  bit0=input_bits + 1  base0=LSB of Input  dbl_ovrd=off  block_type=slice
  Slice7 : xbsIndex_r4/Slice  nbits=5-1  boolean_output=off  mode=Two Bit Locations  bit1=-1  base1=MSB of Input  bit0=0  base0=LSB of Input  dbl_ovrd=off  block_type=slice
  Slice8 : xbsIndex_r4/Slice  nbits=5-1  boolean_output=on  mode=Upper Bit Location + Width  bit1=0  base1=MSB of Input  bit0=0  base0=LSB of Input  dbl_ovrd=off  block_type=slice
  Terminator2 : Terminator
  Terminator3 : Terminator
  Terminator4 : Terminator
  d0 : xbsIndex_r4/Register  init=0  rst=on  en=on  dbl_ovrd=off  block_type=register
  edge_detect1 : Subsystem  AncestorBlock=casper_library_misc/edge_detect  mask(edge_detect){edge=Falling, polarity=Active High, x_in=[0 0.08 0.08 0.16 0.16 0.24 0.24 0.32 0.32 0.4], y_in=[-1 -1  1  1  1  1  1  1  1  1], x_out=[0.6 0.68 0.68 0.76 0.76 0.84 0.84 0.92 0.92 1], y_out=[-1 -1  1  1 -1 -1 -1 -1 -1 -1]}
      mask prompts: edge "Edge Type"; polarity "Output Polarity"; x_in "Input X Positions"; y_in "Input Y Positions"; x_out "Output X Positions"; y_out "Output Y Positions"
      mask help: Output is active for one-cycle after each edge of the specified type (i.e. rising, falling or both).
      mask init: same as snb_d/edge_detect1
      settings: AttributesFormatString=|
      | falling edges
      | active high
      mask Help: Output is active for one-cycle after each edge of the specified type (i.e. rising, falling, or both).  Latency is zero.
      mask TypeOptions edge: Rising | Falling | Both
      mask TypeOptions polarity: Active High | Active Low
      mask Display:
      | plot(x_in_num,0.5+y_in_num*0.2);
      | plot(x_out_num,0.5+y_out_num*0.2);
  edge_detect2 : Subsystem  AncestorBlock=casper_library_misc/edge_detect  mask(edge_detect){edge=Falling, polarity=Active High, x_in=[0 0.08 0.08 0.16 0.16 0.24 0.24 0.32 0.32 0.4], y_in=[-1 -1  1  1  1  1  1  1  1  1], x_out=[0.6 0.68 0.68 0.76 0.76 0.84 0.84 0.92 0.92 1], y_out=[-1 -1  1  1 -1 -1 -1 -1 -1 -1]}
      mask prompts: edge "Edge Type"; polarity "Output Polarity"; x_in "Input X Positions"; y_in "Input Y Positions"; x_out "Output X Positions"; y_out "Output Y Positions"
      mask help: Output is active for one-cycle after each edge of the specified type (i.e. rising, falling or both).
      mask init: same as snb_d/edge_detect1
      settings: AttributesFormatString=|
      | falling edges
      | active high
      mask Help: Output is active for one-cycle after each edge of the specified type (i.e. rising, falling, or both).  Latency is zero.
      mask TypeOptions edge: Rising | Falling | Both
      mask TypeOptions polarity: Active High | Active Low
      mask Display:
      | plot(x_in_num,0.5+y_in_num*0.2);
      | plot(x_out_num,0.5+y_out_num*0.2);
  edge_detect3 : Subsystem  AncestorBlock=casper_library_misc/edge_detect  mask(edge_detect){edge=Falling, polarity=Active High, x_in=[0 0.08 0.08 0.16 0.16 0.24 0.24 0.32 0.32 0.4], y_in=[-1 -1  1  1  1  1  1  1  1  1], x_out=[0.6 0.68 0.68 0.76 0.76 0.84 0.84 0.92 0.92 1], y_out=[-1 -1  1  1 -1 -1 -1 -1 -1 -1]}
      mask prompts: edge "Edge Type"; polarity "Output Polarity"; x_in "Input X Positions"; y_in "Input Y Positions"; x_out "Output X Positions"; y_out "Output Y Positions"
      mask help: Output is active for one-cycle after each edge of the specified type (i.e. rising, falling or both).
      mask init: same as snb_d/edge_detect1
      settings: AttributesFormatString=|
      | falling edges
      | active high
      mask Help: Output is active for one-cycle after each edge of the specified type (i.e. rising, falling, or both).  Latency is zero.
      mask TypeOptions edge: Rising | Falling | Both
      mask TypeOptions polarity: Active High | Active Low
      mask Display:
      | plot(x_in_num,0.5+y_in_num*0.2);
      | plot(x_out_num,0.5+y_out_num*0.2);
  edge_detect5 : Subsystem  AncestorBlock=casper_library_misc/edge_detect  mask(edge_detect){edge=Falling, polarity=Active High, x_in=[0 0.08 0.08 0.16 0.16 0.24 0.24 0.32 0.32 0.4], y_in=[-1 -1  1  1  1  1  1  1  1  1], x_out=[0.6 0.68 0.68 0.76 0.76 0.84 0.84 0.92 0.92 1], y_out=[-1 -1  1  1 -1 -1 -1 -1 -1 -1]}
      mask prompts: edge "Edge Type"; polarity "Output Polarity"; x_in "Input X Positions"; y_in "Input Y Positions"; x_out "Output X Positions"; y_out "Output Y Positions"
      mask help: Output is active for one-cycle after each edge of the specified type (i.e. rising, falling or both).
      mask init: same as snb_d/edge_detect1
      settings: AttributesFormatString=|
      | falling edges
      | active high
      mask Help: Output is active for one-cycle after each edge of the specified type (i.e. rising, falling, or both).  Latency is zero.
      mask TypeOptions edge: Rising | Falling | Both
      mask TypeOptions polarity: Active High | Active Low
      mask Display:
      | plot(x_in_num,0.5+y_in_num*0.2);
      | plot(x_out_num,0.5+y_out_num*0.2);
  in : xbsIndex_r4/WaveScope  block_type=wavescope
      settings: block_version=11.4
  ind_trig : xbsIndex_r4/Register  init=0  rst=on  en=on  dbl_ovrd=off  block_type=register
  ind_trig1 : xbsIndex_r4/Register  init=0  rst=on  en=on  dbl_ovrd=off  block_type=register
  out : xbsIndex_r4/WaveScope  block_type=wavescope
      settings: block_version=11.4
  pause_arm : xbsIndex_r4/Register  init=0  rst=on  en=on  dbl_ovrd=off  block_type=register
  pause_ctr : xbsIndex_r4/Counter  cnt_type=Free Running  cnt_to=Inf  operation=Up  start_count=0  cnt_by_val=1  arith_type=Unsigned  n_bits=pause_bits  bin_pt=0  load_pin=off  rst=on  en=on  explicit_period=on  period=1  dbl_ovrd=off  use_behavioral_HDL=off  implementation=Fabric  use_rpm=off  block_type=counter
  qdr : Subsystem  Tag=xps:qdr  AncestorBlock=xps_library/qdr  mask(qdr){which_qdr=qdr0, qdr_awidth=16, use_sniffer=on}
      mask prompts: which_qdr "QDR Chip"; qdr_awidth "Simulation QDR address width"; use_sniffer "Include CPU Interface"
      mask help:
      | Interface to the QDR II SRAM device on ROACH and ROACH2.
      | For ROACH, use only QDR chips qdr0 or qdr1.
      | For ROACH2, use qdr chips qdr0, qdr1, qdr2 or qdr3.
      mask init:
      | qdr_mask(gcb);
      mask TypeOptions which_qdr: qdr0 | qdr1 | qdr2 | qdr3
  qdr_addr_ctr : xbsIndex_r4/Counter  cnt_type=Free Running  cnt_to=Inf  operation=Up  start_count=0  cnt_by_val=2^(input_bits-1)  arith_type=Unsigned  n_bits=input_bits + ct_bits - 1  bin_pt=0  load_pin=off  rst=on  en=on  explicit_period=on  period=1  dbl_ovrd=off  use_behavioral_HDL=off  implementation=Fabric  use_rpm=off  block_type=counter
  qdr_scope : xbsIndex_r4/WaveScope  block_type=wavescope
      settings: block_version=11.4
  read_arm_main : xbsIndex_r4/Register  init=0  rst=on  en=on  dbl_ovrd=off  block_type=register
  read_ctr : xbsIndex_r4/Counter  cnt_type=Free Running  cnt_to=Inf  operation=Up  start_count=0  cnt_by_val=1  arith_type=Unsigned  n_bits=input_bits + ct_bits + 1  bin_pt=0  load_pin=off  rst=on  en=on  explicit_period=on  period=1  dbl_ovrd=off  use_behavioral_HDL=off  implementation=Fabric  use_rpm=off  block_type=counter
  read_cycle_arm : xbsIndex_r4/Register  init=0  rst=on  en=on  dbl_ovrd=off  block_type=register
  sync_arm : xbsIndex_r4/Register  init=0  rst=on  en=on  dbl_ovrd=off  block_type=register
  wr_addr_ctr : xbsIndex_r4/Counter  cnt_type=Free Running  cnt_to=Inf  operation=Up  start_count=0  cnt_by_val=1  arith_type=Unsigned  n_bits=input_bits + ct_bits  bin_pt=0  load_pin=off  rst=on  en=on  explicit_period=on  period=1  dbl_ovrd=off  use_behavioral_HDL=off  implementation=Fabric  use_rpm=off  block_type=counter
  out_sync : Outport
  out_dv : Outport  Port=2
  out_data72 : Outport  Port=3
  out_addr_error : Outport  Port=4
  wires:
  edge_detect2/1(out) -> read_cycle_arm/3, read_cycle_arm/1, Logical4/1  "rstart"
  [rallow] -> Logical5/2
  [in_data64] -> d0/1
  Slice2/1 -> edge_detect2/1(in)
  Inverter/1 -> Logical5/4
  Slice3/1 -> edge_detect3/1(in)
  Logical5/1 -> [ren]  "ren"
  [waddr] -> Slice2/1
  Delay2/1 -> Logical3/3
  Slice5/1 -> edge_detect5/1(in)
  Logical1/1 -> wr_addr_ctr/2, [wen]  "wen"
  edge_detect5/1(out) -> [rcdone]  "cycle_done"
  Logical4/1 -> [rcen]  "rcycle"
  Slice7/1 -> Slice11/1, Slice12/1, Slice10/1, Slice5/1, Slice4/1, Slice1/1
  Slice8/1 -> [read_bank]  "read_bank"
  read_ctr/1 -> Slice8/1, Slice7/1  "read_ctr"
  [pause_done] -> pause_arm/2
  edge_detect1/1(out) -> [pkt_done]  "pkt_done"
  ct_reset/1 -> [ct_reset]
  [rcen] -> Logical5/1
  [wen] -> Logical7/2
  pause_arm/1 -> [pkt_pause]  "pkt_pause"
  [in_dv] -> Logical1/2, ind_trig/3, d0/3
  [in_sync] -> read_arm_main/2
  [ren] -> Logical7/1
  Logical3/1 -> [rallow]  "rallow"
  edge_detect3/1(out) -> [pause_done], pause_ctr/1  "pause_over"
  pause_ctr/1 -> Slice3/1  "pause_ctr"
  [wen] -> read_arm_main/1, read_arm_main/3
  Logical7/1 -> out_addr_error/1  "addr_error"
  wr_addr_ctr/1 -> [waddr]  "waddr"
  Logical2/1 -> read_cycle_arm/2
  [rarm] -> Logical5/3
  [pkt_pause] -> pause_ctr/2
  Delay3/1 -> Logical3/4
  Constant2/1 -> ind_trig/1
  [wen] -> Delay1/1, Delay2/1, Delay3/1, Delay/1
  [ren] -> read_ctr/2
  Logical6/1 -> [rarm]  "rarm"
  Delay1/1 -> Logical3/2
  sync_arm/1 -> Logical6/1
  Logical/1 -> ind_trig/2
  [in_sync] -> d0/2
  [pkt_pause] -> Inverter/1
  Delay/1 -> Logical3/1
  Slice1/1 -> edge_detect1/1(in)
  [in_sync] -> sync_arm/3, sync_arm/1
  [ct_reset] -> sync_arm/2
  [in_sync] -> read_ctr/1
  [pkt_done] -> pause_arm/3, pause_arm/1
  read_arm_main/1 -> Logical6/2
  [in_sync] -> wr_addr_ctr/1
  [in_sync] -> Logical/2
  read_cycle_arm/1 -> Logical4/2  "read_cycle_arm"
  ind_trig/1 -> Logical1/1  "ind_trig"
  d0/1 -> [wdata]  "wdata"
  [wen] -> Logical/1
  in_sync/1 -> [in_sync]  "in_sync"
  in_dv/1 -> [in_dv]  "in_dv"
  in_data64/1 -> [in_data64]  "in_data"
  [rcdone] -> Logical2/2
  [in_sync] -> Logical2/1
  Slice10/1 -> [word_sel]  "word_sel"
  Slice11/1 -> Concat2/2
  Slice12/1 -> [cycle_ctr], Concat2/1  "cycle_ctr"
  Concat2/1 -> [read_addr]  "read_addr"
  [in_sync] -> qdr_addr_ctr/1
  [ren] -> qdr_addr_ctr/2
  qdr_addr_ctr/1 -> AddSub/1  "qdr_addr"
  Constant/1 -> Concat3/2
  Concat3/1 -> AddSub/2
  AddSub/1 -> AddSub1/1
  [cycle_ctr] -> AddSub1/2
  AddSub1/1 -> Concat4/2  "qdr_addr_full"
  Slice4/1 -> [pkt_ctr]  "pkt_ctr"
  [pkt_ctr] -> Concat3/1
  Delay8/1 -> Delay19/1, qdr/1(rd_en)  "rden"
  Delay7/1 -> Mux1/2
  [word_sel] -> Delay5/1
  [wen] -> Delay9/1
  qdr/1(data_out) -> [qdr_word]  "dout"
  Mux2/1 -> Logical8/2
  qdr/2(data_valid) -> [qdr_dv]  "dv"
  Constant5/1 -> qdr/3(be)
  Delay16/1 -> Mux1/3
  [wdata] -> Delay15/1
  Mux1/1 -> qdr/4(address)  "addr"
  qdr/5(cal_fail) -> Terminator4/1
  Delay6/1 -> Mux1/1
  Delay9/1 -> qdr/2(wr_en)  "wren"
  qdr/3(ack) -> Terminator2/1
  [qdr_word] -> Delay18/1
  Delay5/1 -> Delay10/1  "wordsel"
  [ren] -> Delay6/1
  [waddr] -> Delay7/1
  [ren] -> Delay8/1
  Delay15/1 -> qdr/5(data_in)  "din"
  Delay14/1 -> Mux2/3  "rendeldel"
  Delay10/1 -> [qdr_phasesel]  "phase_sel"
  qdr/4(phy_ready) -> Terminator3/1
  [qdr_addr_interleave] -> Delay16/1
  Concat4/1 -> [qdr_addr_interleave]
  [read_bank] -> Concat4/1
  [in_sync] -> ind_trig1/3, ind_trig1/1
  ind_trig1/1 -> Logical9/1
  Logical9/1 -> out_sync/1, Logical10/1, ind_trig1/2  "sync_out"
  Delay17/1 -> Logical10/2  "dvout"
  Delay18/1 -> out_data72/1  "dout"
  Delay19/1 -> [ren_delayed]  "ren_del"
  [ren_delayed] -> Mux2/2, Delay14/1
  [qdr_dv] -> Logical8/1
  [qdr_phasesel] -> Mux2/1
  Logical8/1 -> Logical9/2, Delay17/1
  Logical10/1 -> out_dv/1  "dvout"
